simulink model "Part_franchissementVAD"  (Simulink 7.5)
settings: Solver=ode45  StartTime=0.0  StopTime=10.0  RelTol=1e-3
settings Model: Creator=paris  LastModifiedBy=paris

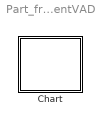
== system Part_franchissementVAD ==
  Chart : Stateflow chart  TreatAsAtomicUnit=on

== stateflow chart Chart ==
  state franchissement VAD
    state Entree
      Virage
      state SV [parallel]
        settings: executionOrder=2
        state SVG
          optim
        state SVD
          optim
      state MANOEUVRES TACTIQUES [parallel]
        settings: executionOrder=1
        state MANOEUVRES ATTENDUES
          state Decelerer : chute vitesse
        state RECUPERATIONS
      state ACTIONS OPERATIONNELLES [parallel]
        settings: executionOrder=3
        state ACTIONS ATTENDUES
          state FreinFluide : frein non nul
            mais pas fort sans rupture
          state VolantFluide : braquage
        state ACTIONS RECUPERATIONS
          state FreinFort
      (default) -> (junction 80) : [ml.progression_SV<>0]
    state Sortie
      Virage
      state SV
        state SVG defaut
        state SVD1
        state SVD
      state MANOEUVRES TACTIQUES
        state MANOEUVRES ATTENDUES
          state Accelerer
          state Redresser
        state RECUPERATIONS
          state freiner
      state ACTIONS OPERATIONNELLES
        state ACTIONS ATTENDUES
          state VolantFluide : contrebraquage
        state Coup de
          volant
        state FREIN
        state ACTIONS RECUPERATIONS
    state Approche
      Virage
      state SVG => optim
    state Fin Gestion
      Courbe
      state ACTIONS OPERATIONNELLES
        state ACTIONS1 ATTENDUES
          state VolantFluide : braquage
        state Coup de
          volant
        state FREIN
        state ACTIONS RECUPERATIONS
      state SV
        state SVG defaut
        state SVD optimisation
        state SVD
      state MANOEUVRES TACTIQUES
        state RECUPERATIONS
          state Tourner brutal
          state Decelerer brutal
        state MANOEUVRES ATTENDUES
          state Tourner
    state Debut Gestion
      Courbe
      state ACTIONS OPERATIONNELLES
        state ACTIONS ATTENDUES
          state FreinFluide : frein non nul
            mais pas fort sans rupture
          state VolantFluide : braquage
        state ACTIONS RECUPERATIONS
        state FreinFort
        state ACTIONS Possibles
          state contrebraquage =
            optimisation
        state FreinTardif
        state Coup de
          volant
      state MANOEUVRES TACTIQUES
        state MANOEUVRES ATTENDUES
          state Tourner
          state Decelerer
        state RECUPERATIONS
          state Tourner brutal
          state Decelerer brutal
      state SV
        state SVG
          defaut
        state SVD
          optilm si piste cyclable
    (default) -> Approche [order 2] : [ml.distPtA<=50]
    Approche -> Entree : [ml.distPtA<=10]
    Entree -> Debut Gestion : [ml.distPtA==0]
    Fin Gestion -> Sortie : [ml.distPtC==0]
    Debut Gestion -> Fin Gestion : [ml.distPtB==0]
    (default) -> (junction 79) [order 1] : [ml.lateralisation_SV==-1]
    (default) -> (junction 81) [order 3] : [ml.lateralisation_SV==1]
  state JUGEMENT ADEQUATION MANOEUVRE SORTIE DE VOIE
    state Sortie Voie Optimisation
    state Sortie Voie Defaut
    state Sortie Voie AUTRE
